simulink model "electricCar230823"  (R2020b)
settings: Solver=FixedStepAuto  StartTime=0.0  StopTime=SIMULPARAM.T_end  FixedStep=SIMULPARAM.Ts  RelTol=1e-3
undefined symbols (not defined in the file or in its folder): BAT, C, CHAp, Currentcontroller, DCM, F, Ki_Current_Con, Kp_Current_Con, Kp_Ucap, Linduc, MTp, RDp, Rinduc, Speedcontroller, T, Uco
libraries: simulink x1
settings Model: Creator=PC  LastModifiedBy=PC

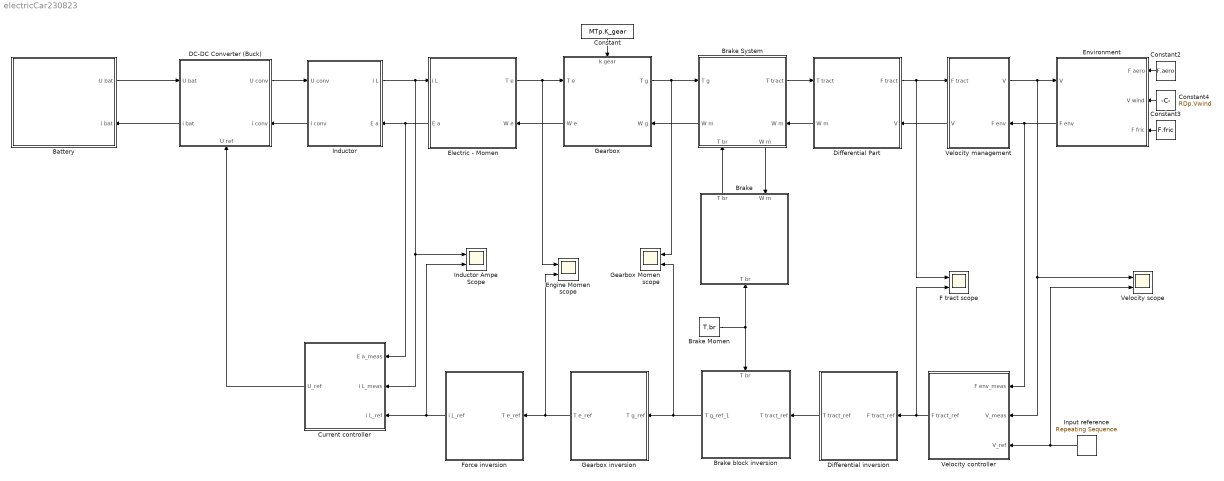
== system electricCar230823 ==
  Battery : Subsystem
      settings: PortSchema="{\"entries\":[{\"content\":{\"sides\":[{\"content\":{\"connectorIds\":[]},\"type\":\"ConnectorPlacement.EquallySpacedRectSide\",\"uuid\":\"1728278d-2efb-45d4-8f99-b2a86feaa846\"},{\"content\":{\"connectorIds\":[\"Out1\",\"In1\"],\"side\":\"RIGHT\"},\"type\":\"ConnectorPlacement.EquallySpacedRectSide\",\"uuid\":\"72e7f82c-4a4c-4bdc-a479-895fa91bb5d6\"},{\"content\":{\"connectorIds\":[],\"side\":\"TOP\"},\"type\":\"ConnectorPlacement.EquallySpacedRectSide\",\"uuid\":\"4ecd59fb-c886-47cd-9c71-6f362398ed11\"},{\"content\":{\"connectorIds\":[],\"side\":\"HIDDEN\"},\"type\":\"ConnectorPlacement.EquallySpacedRectSide\",\"uuid\":\"481497fe-ed83-4130-bda0-6381f15eb2c9\"}]},\"type\":\"ConnectorPlacement.EquallySpacedConnector\",\"uuid\":\"ea3c396a-3ef7-43d2-bef5-b2521c5226f8\"}],\"packageUris\":[\"http://schema.mathworks.com/mf0/Connector/R2020b\"],\"version\":\"1.0\"}"
      mask Display:
      | plot(0,0,100,100, 1.2*[50,57.68,60.77,63.08,64.97,66.58,68,69.26,70.4, 	71.42,72.36,78.28,80,78.28,72.36,71.42,70.4, 	69.26,68,66.58,64.97,63.08,60.77,57.68,50,42.32, 	39.23,36.92,35.03,33.42,32,30.74,29.6,28.58, 	27.64,21.72,20,21.72,27.64,28.58,29.6,30.74,32, 	33.42,35.03,36.92,39.23,42.32,50]-10, 1.2*[20,21,22,23,24,25,26,27,28,29,30,40,50,60,70,71,72, 	73,74,75,76,77,78,79,80,79,78,77,76,75,74,73,72, 	71,70,60,50,40,30,29,28,27,26,25,24,23,22,21,20]-10)
      | disp('ES')
  Brake : Subsystem
      settings: PortSchema="{\"entries\":[{\"content\":{\"sides\":[{\"content\":{\"connectorIds\":[\"In1\",\"Out1\"]},\"type\":\"ConnectorPlacement.EquallySpacedRectSide\",\"uuid\":\"1728278d-2efb-45d4-8f99-b2a86feaa846\"},{\"content\":{\"connectorIds\":[\"In2\"],\"side\":\"RIGHT\"},\"type\":\"ConnectorPlacement.EquallySpacedRectSide\",\"uuid\":\"72e7f82c-4a4c-4bdc-a479-895fa91bb5d6\"},{\"content\":{\"connectorIds\":[],\"side\":\"TOP\"},\"type\":\"ConnectorPlacement.EquallySpacedRectSide\",\"uuid\":\"4ecd59fb-c886-47cd-9c71-6f362398ed11\"},{\"content\":{\"connectorIds\":[],\"side\":\"HIDDEN\"},\"type\":\"ConnectorPlacement.EquallySpacedRectSide\",\"uuid\":\"481497fe-ed83-4130-bda0-6381f15eb2c9\"}]},\"type\":\"ConnectorPlacement.EquallySpacedConnector\",\"uuid\":\"ea3c396a-3ef7-43d2-bef5-b2521c5226f8\"}],\"packageUris\":[\"http://schema.mathworks.com/mf0/Connector/R2020b\"],\"version\":\"1.0\"}"
      mask Display:
      | plot(0,0,100,100, 1.2*[50,57.68,60.77,63.08,64.97,66.58,68,69.26,70.4, 	71.42,72.36,78.28,80,78.28,72.36,71.42,70.4, 	69.26,68,66.58,64.97,63.08,60.77,57.68,50,42.32, 	39.23,36.92,35.03,33.42,32,30.74,29.6,28.58, 	27.64,21.72,20,21.72,27.64,28.58,29.6,30.74,32, 	33.42,35.03,36.92,39.23,42.32,50]-10, 1.2*[20,21,22,23,24,25,26,27,28,29,30,40,50,60,70,71,72, 	73,74,75,76,77,78,79,80,79,78,77,76,75,74,73,72, 	71,70,60,50,40,30,29,28,27,26,25,24,23,22,21,20]-10)
      | disp('MS')
  Brake Momen : Constant  Value=T.br
  Brake System : Subsystem  mask(CM){}
      settings: PortSchema="{\"entries\":[{\"content\":{\"sides\":[{\"content\":{\"connectorIds\":[\"In1\",\"Out3\"]},\"type\":\"ConnectorPlacement.EquallySpacedRectSide\",\"uuid\":\"62bc74ff-9f0a-435b-bbdb-72403e9cc1db\"},{\"content\":{\"connectorIds\":[\"Out1\",\"In3\"],\"side\":\"RIGHT\"},\"type\":\"ConnectorPlacement.EquallySpacedRectSide\",\"uuid\":\"e16e9817-8001-4871-9942-49d69e9da80f\"},{\"content\":{\"connectorIds\":[],\"side\":\"TOP\"},\"type\":\"ConnectorPlacement.EquallySpacedRectSide\",\"uuid\":\"0e99ecee-f353-402b-98e6-e62629e3b5c0\"},{\"content\":{\"connectorIds\":[\"In2\",\"Out2\"],\"side\":\"BOTTOM\"},\"type\":\"ConnectorPlacement.EquallySpacedRectSide\",\"uuid\":\"3f9b191f-4efa-4e46-9672-1631f2ad3889\"},{\"content\":{\"connectorIds\":[],\"side\":\"HIDDEN\"},\"type\":\"ConnectorPlacement.EquallySpacedRectSide\",\"uuid\":\"eab2a9d2-f7eb-47b5-b573-a1d51d411443\"}]},\"type\":\"ConnectorPlacement.EquallySpacedConnector\",\"uuid\":\"edb337c0-73db-4b78-b52e-7735544c1492\"}],\"packageUris\":[\"http://schema.mathworks.com/mf0/Connector/R2020b\"],\"version\":\"1.0\"}"
      mask Display: plot(0,0,100,100,[35,35,95,95,35],[65,10,10,65,65], [5,5,65,65,5],[90,35,35,90,90])
  "Brake block inversion " : Subsystem
      settings: PortSchema="{\"entries\":[{\"content\":{\"sides\":[{\"content\":{\"connectorIds\":[\"In1\"]},\"type\":\"ConnectorPlacement.EquallySpacedRectSide\",\"uuid\":\"730055a7-c930-4640-a945-75cf3ba3ff6f\"},{\"content\":{\"connectorIds\":[\"Out1\"],\"side\":\"RIGHT\"},\"type\":\"ConnectorPlacement.EquallySpacedRectSide\",\"uuid\":\"ff5124cd-06d0-417f-b0e4-eab59cd93227\"},{\"content\":{\"connectorIds\":[\"In2\"],\"side\":\"TOP\"},\"type\":\"ConnectorPlacement.EquallySpacedRectSide\",\"uuid\":\"dac7e156-045e-4392-b76a-344f17dcf5dc\"},{\"content\":{\"connectorIds\":[],\"side\":\"HIDDEN\"},\"type\":\"ConnectorPlacement.EquallySpacedRectSide\",\"uuid\":\"42e29ba6-0723-44e9-ba7d-78428fe859ea\"}]},\"type\":\"ConnectorPlacement.EquallySpacedConnector\",\"uuid\":\"81c30e31-29e4-493d-8a58-533eb4e50f51\"}],\"packageUris\":[\"http://schema.mathworks.com/mf0/Connector/R2020b\"],\"version\":\"1.0\"}"
      mask Display: plot(0,0,100,100,[20,40,100,80,20],[75,20,20,75,75], [0,20,80,60,0],[85,30,30,85,85])
  Constant : Constant  Value=MTp.K_gear
  Constant2 : Constant  Value=F.aero
  Constant3 : Constant  Value=F.fric
  Constant4 : Constant  Value=RDp.Vwind
  Current controller : Subsystem
      mask Display: plot(0,0,100,100, [10,30,90,70,10,90],[90,10,10,90,90,10])
  DC-DC Converter (Buck) : Subsystem
      settings: PortSchema="{\"entries\":[{\"content\":{\"sides\":[{\"content\":{\"connectorIds\":[\"In1\",\"Out2\"]},\"type\":\"ConnectorPlacement.EquallySpacedRectSide\",\"uuid\":\"f2e25d2c-aa7f-4861-8c3a-38af6928b037\"},{\"content\":{\"connectorIds\":[\"Out1\",\"In3\"],\"side\":\"RIGHT\"},\"type\":\"ConnectorPlacement.EquallySpacedRectSide\",\"uuid\":\"82b8127f-d667-4684-9845-8beb7a647838\"},{\"content\":{\"connectorIds\":[],\"side\":\"TOP\"},\"type\":\"ConnectorPlacement.EquallySpacedRectSide\",\"uuid\":\"76c3910b-3260-4deb-ab83-4fcb3794542a\"},{\"content\":{\"connectorIds\":[\"In2\"],\"side\":\"BOTTOM\"},\"type\":\"ConnectorPlacement.EquallySpacedRectSide\",\"uuid\":\"340d5235-774f-48d9-bcc2-670650272594\"},{\"content\":{\"connectorIds\":[],\"side\":\"HIDDEN\"},\"type\":\"ConnectorPlacement.EquallySpacedRectSide\",\"uuid\":\"3b8b73f1-b23a-4cba-8ed6-bcf75c8f378e\"}]},\"type\":\"ConnectorPlacement.EquallySpacedConnector\",\"uuid\":\"8076e3c1-f844-447c-82cb-af3927bb8eb4\"}],\"packageUris\":[\"http://schema.mathworks.com/mf0/Connector/R2020b\"],\"version\":\"1.0\"}"
  Differential Part : Subsystem
      settings: PortSchema="{\"entries\":[{\"content\":{\"sides\":[{\"content\":{\"connectorIds\":[\"In1\",\"Out2\"]},\"type\":\"ConnectorPlacement.EquallySpacedRectSide\",\"uuid\":\"b394e922-8364-4918-bac2-7f5831442eb0\"},{\"content\":{\"connectorIds\":[\"Out1\",\"In2\"],\"side\":\"RIGHT\"},\"type\":\"ConnectorPlacement.EquallySpacedRectSide\",\"uuid\":\"e0445a5e-fdf7-4c21-a205-54d904cb27ed\"},{\"content\":{\"connectorIds\":[],\"side\":\"TOP\"},\"type\":\"ConnectorPlacement.EquallySpacedRectSide\",\"uuid\":\"c34109ca-a85d-4763-b4ce-c9c887f4fb15\"},{\"content\":{\"connectorIds\":[],\"side\":\"HIDDEN\"},\"type\":\"ConnectorPlacement.EquallySpacedRectSide\",\"uuid\":\"2368fea2-69ff-4966-ae44-ff953213b5b6\"}]},\"type\":\"ConnectorPlacement.EquallySpacedConnector\",\"uuid\":\"11143b87-4d9b-4f42-a2c1-62596b1f3291\"}],\"packageUris\":[\"http://schema.mathworks.com/mf0/Connector/R2020b\"],\"version\":\"1.0\"}"
      mask Display: plot(0,0,100,100, 1.4*[50,57.68,60.77,63.08,64.97,66.58,68,69.26,70.4, 	71.42,72.36,78.28,80,78.28,72.36,71.42,70.4, 	69.26,68,66.58,64.97,63.08,60.77,57.68,50,42.32, 	39.23,36.92,35.03,33.42,32,30.74,29.6,28.58, 	27.64,21.72,20,21.72,27.64,28.58,29.6,30.74,32, 	33.42,35.03,36.92,39.23,42.32,50]-20, 1.4*[20,21,22,23,24,25,26,27,28,29,30,40,50,60,70,71,72, 	73,74,75,76,77,78,79,80,79,78,77,76,75,74,73,72, 	71,70,60,50,40,30,29,28,27,26,25,24,23,22,21,20]-20)
  Differential inversion : Subsystem
      mask Display: plot(0,0,100,100,[10,30,90,70,10],[90,10,10,90,90])
  Electric - Momen : Subsystem
      settings: PortSchema="{\"entries\":[{\"content\":{\"sides\":[{\"content\":{\"connectorIds\":[\"In1\",\"Out2\"]},\"type\":\"ConnectorPlacement.EquallySpacedRectSide\",\"uuid\":\"b394e922-8364-4918-bac2-7f5831442eb0\"},{\"content\":{\"connectorIds\":[\"Out1\",\"In2\"],\"side\":\"RIGHT\"},\"type\":\"ConnectorPlacement.EquallySpacedRectSide\",\"uuid\":\"e0445a5e-fdf7-4c21-a205-54d904cb27ed\"},{\"content\":{\"connectorIds\":[],\"side\":\"TOP\"},\"type\":\"ConnectorPlacement.EquallySpacedRectSide\",\"uuid\":\"c34109ca-a85d-4763-b4ce-c9c887f4fb15\"},{\"content\":{\"connectorIds\":[],\"side\":\"HIDDEN\"},\"type\":\"ConnectorPlacement.EquallySpacedRectSide\",\"uuid\":\"2368fea2-69ff-4966-ae44-ff953213b5b6\"}]},\"type\":\"ConnectorPlacement.EquallySpacedConnector\",\"uuid\":\"11143b87-4d9b-4f42-a2c1-62596b1f3291\"}],\"packageUris\":[\"http://schema.mathworks.com/mf0/Connector/R2020b\"],\"version\":\"1.0\"}"
      mask Display: plot(0,0,100,100, 1.4*[50,57.68,60.77,63.08,64.97,66.58,68,69.26,70.4, 	71.42,72.36,78.28,80,78.28,72.36,71.42,70.4, 	69.26,68,66.58,64.97,63.08,60.77,57.68,50,42.32, 	39.23,36.92,35.03,33.42,32,30.74,29.6,28.58, 	27.64,21.72,20,21.72,27.64,28.58,29.6,30.74,32, 	33.42,35.03,36.92,39.23,42.32,50]-20, 1.4*[20,21,22,23,24,25,26,27,28,29,30,40,50,60,70,71,72, 	73,74,75,76,77,78,79,80,79,78,77,76,75,74,73,72, 	71,70,60,50,40,30,29,28,27,26,25,24,23,22,21,20]-20)
  Engine Momen scope : Scope  NumInputPorts=2
  Environment : Subsystem
      settings: PortSchema="{\"entries\":[{\"content\":{\"sides\":[{\"content\":{\"connectorIds\":[\"In1\",\"Out1\"]},\"type\":\"ConnectorPlacement.EquallySpacedRectSide\",\"uuid\":\"1728278d-2efb-45d4-8f99-b2a86feaa846\"},{\"content\":{\"connectorIds\":[\"In2\",\"In3\",\"In4\"],\"side\":\"RIGHT\"},\"type\":\"ConnectorPlacement.EquallySpacedRectSide\",\"uuid\":\"72e7f82c-4a4c-4bdc-a479-895fa91bb5d6\"},{\"content\":{\"connectorIds\":[],\"side\":\"TOP\"},\"type\":\"ConnectorPlacement.EquallySpacedRectSide\",\"uuid\":\"4ecd59fb-c886-47cd-9c71-6f362398ed11\"},{\"content\":{\"connectorIds\":[],\"side\":\"BOTTOM\"},\"type\":\"ConnectorPlacement.EquallySpacedRectSide\",\"uuid\":\"f99f3cdf-333c-494c-9d28-40c67ff9c903\"},{\"content\":{\"connectorIds\":[],\"side\":\"HIDDEN\"},\"type\":\"ConnectorPlacement.EquallySpacedRectSide\",\"uuid\":\"481497fe-ed83-4130-bda0-6381f15eb2c9\"}]},\"type\":\"ConnectorPlacement.EquallySpacedConnector\",\"uuid\":\"ea3c396a-3ef7-43d2-bef5-b2521c5226f8\"}],\"packageUris\":[\"http://schema.mathworks.com/mf0/Connector/R2020b\"],\"version\":\"1.0\"}"
      mask Display:
      | plot(0,0,100,100, 1.2*[50,57.68,60.77,63.08,64.97,66.58,68,69.26,70.4, 	71.42,72.36,78.28,80,78.28,72.36,71.42,70.4, 	69.26,68,66.58,64.97,63.08,60.77,57.68,50,42.32, 	39.23,36.92,35.03,33.42,32,30.74,29.6,28.58, 	27.64,21.72,20,21.72,27.64,28.58,29.6,30.74,32, 	33.42,35.03,36.92,39.23,42.32,50]-10, 1.2*[20,21,22,23,24,25,26,27,28,29,30,40,50,60,70,71,72, 	73,74,75,76,77,78,79,80,79,78,77,76,75,74,73,72, 	71,70,60,50,40,30,29,28,27,26,25,24,23,22,21,20]-10)
      | disp('MS')
  F tract scope : Scope  NumInputPorts=2
  Force inversion : Subsystem
      mask Display: plot(0,0,100,100,[10,30,90,70,10],[90,10,10,90,90])
  Gearbox : Subsystem  mask(Hacheur){}
      settings: PortSchema="{\"entries\":[{\"content\":{\"sides\":[{\"content\":{\"connectorIds\":[\"In1\",\"Out2\"]},\"type\":\"ConnectorPlacement.EquallySpacedRectSide\",\"uuid\":\"d88878b3-8f90-4ef1-90e8-2bd7cd7a4565\"},{\"content\":{\"connectorIds\":[\"Out1\",\"In3\"],\"side\":\"RIGHT\"},\"type\":\"ConnectorPlacement.EquallySpacedRectSide\",\"uuid\":\"d9733dfd-1e25-499b-80f7-04f083537083\"},{\"content\":{\"connectorIds\":[\"In2\"],\"side\":\"TOP\"},\"type\":\"ConnectorPlacement.EquallySpacedRectSide\",\"uuid\":\"7063ddce-722e-4bc9-ac26-cf4ab5e61559\"},{\"content\":{\"connectorIds\":[],\"side\":\"BOTTOM\"},\"type\":\"ConnectorPlacement.EquallySpacedRectSide\",\"uuid\":\"2850ab80-1d34-4652-9b8a-8e0e6fbc5749\"},{\"content\":{\"connectorIds\":[],\"side\":\"HIDDEN\"},\"type\":\"ConnectorPlacement.EquallySpacedRectSide\",\"uuid\":\"288ff06e-21e8-474f-a776-208acbd15993\"}]},\"type\":\"ConnectorPlacement.EquallySpacedConnector\",\"uuid\":\"1890fa73-b710-46d0-95bc-083b3bceb9fd\"}],\"packageUris\":[\"http://schema.mathworks.com/mf0/Connector/R2020b\"],\"version\":\"1.0\"}"
      mask Display: plot(0,0,100,100,[10,10,90,90,10],[90,10,10,90,90])
  Gearbox Momen scope : Scope  NumInputPorts=2
  Gearbox inversion : Subsystem
      mask Display: plot(0,0,100,100,[10,30,90,70,10],[90,10,10,90,90])
  Inductor : Subsystem  mask(CM){}
      settings: PortSchema="{\"entries\":[{\"content\":{\"sides\":[{\"content\":{\"connectorIds\":[\"In1\",\"Out2\"]},\"type\":\"ConnectorPlacement.EquallySpacedRectSide\",\"uuid\":\"b394e922-8364-4918-bac2-7f5831442eb0\"},{\"content\":{\"connectorIds\":[\"Out1\",\"In2\"],\"side\":\"RIGHT\"},\"type\":\"ConnectorPlacement.EquallySpacedRectSide\",\"uuid\":\"e0445a5e-fdf7-4c21-a205-54d904cb27ed\"},{\"content\":{\"connectorIds\":[],\"side\":\"TOP\"},\"type\":\"ConnectorPlacement.EquallySpacedRectSide\",\"uuid\":\"c34109ca-a85d-4763-b4ce-c9c887f4fb15\"},{\"content\":{\"connectorIds\":[],\"side\":\"HIDDEN\"},\"type\":\"ConnectorPlacement.EquallySpacedRectSide\",\"uuid\":\"2368fea2-69ff-4966-ae44-ff953213b5b6\"}]},\"type\":\"ConnectorPlacement.EquallySpacedConnector\",\"uuid\":\"11143b87-4d9b-4f42-a2c1-62596b1f3291\"}],\"packageUris\":[\"http://schema.mathworks.com/mf0/Connector/R2020b\"],\"version\":\"1.0\"}"
      mask Display: plot(0,0,100,100,[10,10,90,90,10],[90,10,10,90,90], [10,90],[10,90])
  Inductor Ampe Scope : Scope  NumInputPorts=2
  Input reference : simulink/Sources/Repeating Sequence  rep_seq_t=[0 5 10 20 50.5 66.5 107.5]  rep_seq_y=[5 0 0 30 40 40*1.5 40*1.5]
  Velocity controller : Subsystem
      mask Display: plot(0,0,100,100, [10,30,90,70,10,90],[90,10,10,90,90,10])
  Velocity management : Subsystem  mask(CM){}
      settings: PortSchema="{\"entries\":[{\"content\":{\"sides\":[{\"content\":{\"connectorIds\":[\"In1\",\"Out2\"]},\"type\":\"ConnectorPlacement.EquallySpacedRectSide\",\"uuid\":\"b394e922-8364-4918-bac2-7f5831442eb0\"},{\"content\":{\"connectorIds\":[\"Out1\",\"In2\"],\"side\":\"RIGHT\"},\"type\":\"ConnectorPlacement.EquallySpacedRectSide\",\"uuid\":\"e0445a5e-fdf7-4c21-a205-54d904cb27ed\"},{\"content\":{\"connectorIds\":[],\"side\":\"TOP\"},\"type\":\"ConnectorPlacement.EquallySpacedRectSide\",\"uuid\":\"c34109ca-a85d-4763-b4ce-c9c887f4fb15\"},{\"content\":{\"connectorIds\":[],\"side\":\"HIDDEN\"},\"type\":\"ConnectorPlacement.EquallySpacedRectSide\",\"uuid\":\"2368fea2-69ff-4966-ae44-ff953213b5b6\"}]},\"type\":\"ConnectorPlacement.EquallySpacedConnector\",\"uuid\":\"11143b87-4d9b-4f42-a2c1-62596b1f3291\"}],\"packageUris\":[\"http://schema.mathworks.com/mf0/Connector/R2020b\"],\"version\":\"1.0\"}"
      mask Display: plot(0,0,100,100,[10,10,90,90,10],[90,10,10,90,90], [10,90],[10,90])
  Velocity scope : Scope  NumInputPorts=2
  wires:
  DC-DC Converter (Buck)/1(U conv) -> Inductor/1(U conv)
  DC-DC Converter (Buck)/2(i bat) -> Battery/1(i bat)
  Constant/1 -> Gearbox/2(k gear)
  Battery/1(U bat) -> DC-DC Converter (Buck)/1(U bat)
  Electric - Momen/2(E a) -> Current controller/1(E a_meas), Inductor/2(E a)
  Inductor/1(i L) -> Inductor Ampe Scope/1, Current controller/2(i L_meas), Electric - Momen/1(i L)
  Gearbox/2(W e) -> Electric - Momen/2(W e)
  Inductor/2(i conv) -> DC-DC Converter (Buck)/3(i conv)
  Electric - Momen/1(T e) -> Engine Momen scope/1, Gearbox/1(T e)
  Brake System/2(W m) -> Brake/1(W m)
  Brake/1("T br ") -> Brake System/2(T br)
  Gearbox/1(T g) -> Brake System/1(T g), Gearbox Momen scope/1
  Brake System/3("W m  ") -> Gearbox/3(W g)
  Velocity management/2(V) -> Differential Part/2(V)
  Differential Part/1(F tract) -> F tract scope/1, Velocity management/1(F tract)
  Brake System/1(T tract) -> Differential Part/1(T tract)
  Differential Part/2(W m) -> Brake System/3("W m ")
  Environment/1(F env) -> Velocity controller/1(F env_meas), Velocity management/2(F env)
  Current controller/1(U_ref) -> DC-DC Converter (Buck)/2(U ref)
  Constant3/1 -> Environment/4(F fric)
  Constant2/1 -> Environment/2(F aero)
  Constant4/1 -> Environment/3(V wind)
  Force inversion/1(i L_ref) -> Inductor Ampe Scope/2, Current controller/3(i L_ref)
  Velocity controller/1(F tract_ref) -> F tract scope/2, Differential inversion/1(F tract_ref)
  Differential inversion/1(T tract_ref) -> "Brake block inversion "/1(T tract_ref)
  "Brake block inversion "/1(T g_ref_1) -> Gearbox Momen scope/2, Gearbox inversion/1(T g_ref)
  Gearbox inversion/1(T e_ref) -> Engine Momen scope/2, Force inversion/1(T e_ref)
  Velocity management/1("V ") -> Environment/1(V), Velocity controller/2(V_meas), Velocity scope/1
  Input reference/1 -> Velocity scope/2, Velocity controller/3(V_ref)
  Brake Momen/1 -> "Brake block inversion "/2(T br), Brake/2(T br)

== system electricCar230823/Battery ==
  i bat : Inport
  Constant : Constant  Value=BAT.U
  Terminator : Terminator
  U bat : Outport  InitialOutput=0
  wires:
  i bat/1 -> Terminator/1
  Constant/1 -> U bat/1

== system electricCar230823/Brake ==
  W m : Inport
  T br : Inport  Port=2
  Terminator : Terminator
  "T br " : Outport  InitialOutput=0
  wires:
  T br/1 -> "T br "/1
  W m/1 -> Terminator/1

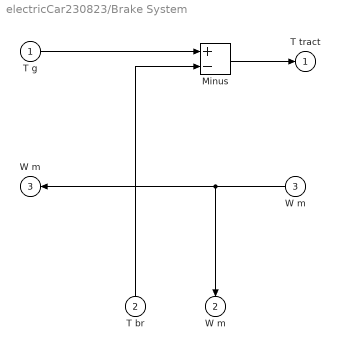
== system electricCar230823/Brake System ==
  T g : Inport
  T br : Inport  Port=2
  "W m " : Inport  Port=3
  Minus : Sum  Inputs=+-
  T tract : Outport  InitialOutput=0
  W m : Outport  Port=2  InitialOutput=0
  "W m  " : Outport  Port=3  InitialOutput=0
  wires:
  T g/1 -> Minus/1
  Minus/1 -> T tract/1
  T br/1 -> Minus/2
  "W m "/1 -> W m/1, "W m  "/1

== system electricCar230823/Brake block inversion  ==
  T tract_ref : Inport
  T br : Inport  Port=2
  Minus : Sum  Inputs=+-
  T g_ref_1 : Outport  InitialOutput=0
  wires:
  T tract_ref/1 -> Minus/1
  T br/1 -> Minus/2
  Minus/1 -> T g_ref_1/1

== system electricCar230823/Current controller ==
  E a_meas : Inport
  i L_meas : Inport  Port=2
  i L_ref : Inport  Port=3
  IP Controller : Subsystem
  PI Controller : Subsystem
  U_ref : Outport  InitialOutput=0
  wires:
  PI Controller/1(U_ref) -> U_ref/1
  i L_meas/1 -> PI Controller/2(i L_meas)
  E a_meas/1 -> PI Controller/1(E a_meas)
  i L_ref/1 -> PI Controller/3(i L_ref)

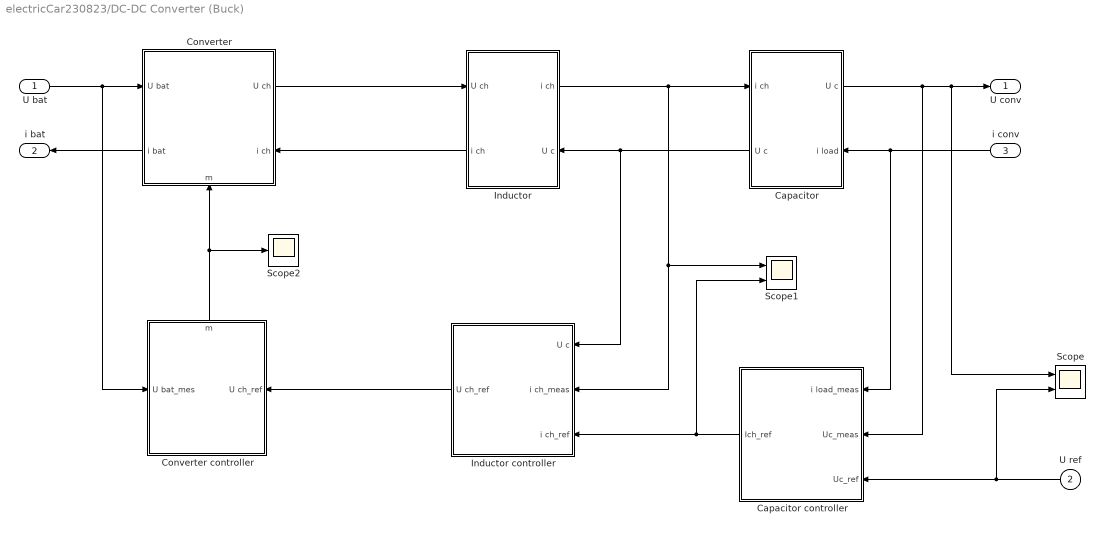
== system electricCar230823/DC-DC Converter (Buck) ==
  U bat : Inport
  U ref : Inport  Port=2
  i conv : Inport  Port=3
  Capacitor : Subsystem  mask(CM){}
      settings: PortSchema="{\"entries\":[{\"content\":{\"sides\":[{\"content\":{\"connectorIds\":[\"In1\",\"Out2\"]},\"type\":\"ConnectorPlacement.EquallySpacedRectSide\",\"uuid\":\"8b9f6a53-b0ce-4fb6-ba22-844cc3c0ad7c\"},{\"content\":{\"connectorIds\":[\"Out1\",\"In2\"],\"side\":\"RIGHT\"},\"type\":\"ConnectorPlacement.EquallySpacedRectSide\",\"uuid\":\"cf1dddcb-91a5-42be-b809-81485d04749f\"},{\"content\":{\"connectorIds\":[],\"side\":\"TOP\"},\"type\":\"ConnectorPlacement.EquallySpacedRectSide\",\"uuid\":\"6b0fe42a-e78b-443e-b09d-31143c938294\"},{\"content\":{\"connectorIds\":[],\"side\":\"HIDDEN\"},\"type\":\"ConnectorPlacement.EquallySpacedRectSide\",\"uuid\":\"92c1545a-c508-44c0-b705-53a96b01068d\"}]},\"type\":\"ConnectorPlacement.EquallySpacedConnector\",\"uuid\":\"979f83f8-9940-4886-be45-d6e0e0e53bbd\"}],\"packageUris\":[\"http://schema.mathworks.com/mf0/Connector/R2020b\"],\"version\":\"1.0\"}"
      mask Display: plot(0,0,100,100,[10,10,90,90,10],[90,10,10,90,90], [10,90],[10,90])
  Capacitor controller : Subsystem
      mask Display: plot(0,0,100,100, [10,30,90,70,10,90],[90,10,10,90,90,10])
  Converter : Subsystem  mask(Hacheur){}
      settings: PortSchema="{\"entries\":[{\"content\":{\"sides\":[{\"content\":{\"connectorIds\":[\"In1\",\"Out2\"]},\"type\":\"ConnectorPlacement.EquallySpacedRectSide\",\"uuid\":\"c60d43d5-6da5-438e-89cb-fd4b71327869\"},{\"content\":{\"connectorIds\":[\"Out1\",\"In3\"],\"side\":\"RIGHT\"},\"type\":\"ConnectorPlacement.EquallySpacedRectSide\",\"uuid\":\"3d284952-b10a-4f69-b6ba-c89d88fd27ff\"},{\"content\":{\"connectorIds\":[],\"side\":\"TOP\"},\"type\":\"ConnectorPlacement.EquallySpacedRectSide\",\"uuid\":\"b76f213b-a89b-4ddb-95af-c15166783b82\"},{\"content\":{\"connectorIds\":[\"In2\"],\"side\":\"BOTTOM\"},\"type\":\"ConnectorPlacement.EquallySpacedRectSide\",\"uuid\":\"5563bba7-a4d6-45e0-a571-46d0680df108\"},{\"content\":{\"connectorIds\":[],\"side\":\"HIDDEN\"},\"type\":\"ConnectorPlacement.EquallySpacedRectSide\",\"uuid\":\"086c2170-6f4c-4142-a25f-314308635861\"}]},\"type\":\"ConnectorPlacement.EquallySpacedConnector\",\"uuid\":\"18a4dcbf-0877-4e56-9ceb-c80d259dd4b7\"}],\"packageUris\":[\"http://schema.mathworks.com/mf0/Connector/R2020b\"],\"version\":\"1.0\"}"
      mask Display: plot(0,0,100,100,[10,10,90,90,10],[90,10,10,90,90])
  Converter controller : Subsystem
      settings: PortSchema="{\"entries\":[{\"content\":{\"sides\":[{\"content\":{\"connectorIds\":[\"In1\"]},\"type\":\"ConnectorPlacement.EquallySpacedRectSide\",\"uuid\":\"badc3caa-6192-4446-bf39-33dbdad74a9c\"},{\"content\":{\"connectorIds\":[\"In2\"],\"side\":\"RIGHT\"},\"type\":\"ConnectorPlacement.EquallySpacedRectSide\",\"uuid\":\"1170bffd-3f0f-42f5-893b-0e18c3005bf1\"},{\"content\":{\"connectorIds\":[\"Out1\"],\"side\":\"TOP\"},\"type\":\"ConnectorPlacement.EquallySpacedRectSide\",\"uuid\":\"7a85b726-b466-447a-a747-1454cd7b1f05\"},{\"content\":{\"connectorIds\":[],\"side\":\"HIDDEN\"},\"type\":\"ConnectorPlacement.EquallySpacedRectSide\",\"uuid\":\"d7fbd796-8c34-4fc1-83a8-47ced3c788b9\"}]},\"type\":\"ConnectorPlacement.EquallySpacedConnector\",\"uuid\":\"74fa73a9-ee93-4918-a076-3243bad27dc9\"}],\"packageUris\":[\"http://schema.mathworks.com/mf0/Connector/R2020b\"],\"version\":\"1.0\"}"
      mask Display: plot(0,0,100,100,[10,30,90,70,10],[90,10,10,90,90])
  Inductor : Subsystem  mask(CM){}
      settings: PortSchema="{\"entries\":[{\"content\":{\"sides\":[{\"content\":{\"connectorIds\":[\"In1\",\"Out2\"]},\"type\":\"ConnectorPlacement.EquallySpacedRectSide\",\"uuid\":\"8b9f6a53-b0ce-4fb6-ba22-844cc3c0ad7c\"},{\"content\":{\"connectorIds\":[\"Out1\",\"In2\"],\"side\":\"RIGHT\"},\"type\":\"ConnectorPlacement.EquallySpacedRectSide\",\"uuid\":\"cf1dddcb-91a5-42be-b809-81485d04749f\"},{\"content\":{\"connectorIds\":[],\"side\":\"TOP\"},\"type\":\"ConnectorPlacement.EquallySpacedRectSide\",\"uuid\":\"6b0fe42a-e78b-443e-b09d-31143c938294\"},{\"content\":{\"connectorIds\":[],\"side\":\"HIDDEN\"},\"type\":\"ConnectorPlacement.EquallySpacedRectSide\",\"uuid\":\"92c1545a-c508-44c0-b705-53a96b01068d\"}]},\"type\":\"ConnectorPlacement.EquallySpacedConnector\",\"uuid\":\"979f83f8-9940-4886-be45-d6e0e0e53bbd\"}],\"packageUris\":[\"http://schema.mathworks.com/mf0/Connector/R2020b\"],\"version\":\"1.0\"}"
      mask Display: plot(0,0,100,100,[10,10,90,90,10],[90,10,10,90,90], [10,90],[10,90])
  Inductor controller : Subsystem
      mask Display: plot(0,0,100,100, [10,30,90,70,10,90],[90,10,10,90,90,10])
  Scope : Scope  NumInputPorts=2
  Scope1 : Scope  NumInputPorts=2
  Scope2 : Scope
  U conv : Outport
  i bat : Outport  Port=2
  wires:
  Capacitor controller/1(Ich_ref) -> Scope1/2, Inductor controller/3(i ch_ref)
  U bat/1 -> Converter controller/2(U bat_mes), Converter/1(U bat)
  Converter controller/1(m) -> Scope2/1, Converter/2(m)
  i conv/1 -> Capacitor controller/1(i load_meas), Capacitor/2(i load)
  U ref/1 -> Scope/2, Capacitor controller/3(Uc_ref)
  Inductor controller/1(U ch_ref) -> Converter controller/1(U ch_ref)
  Converter/1(U ch) -> Inductor/1(U ch)
  Capacitor/1("U c ") -> Capacitor controller/2(Uc_meas), U conv/1, Scope/1
  Converter/2(i bat) -> i bat/1
  Capacitor/2(U c) -> Inductor controller/1(U c), Inductor/2(U c)
  Inductor/2("i ch ") -> Converter/3(i ch)
  Inductor/1(i ch) -> Inductor controller/2(i ch_meas), Scope1/1, Capacitor/1(i ch)

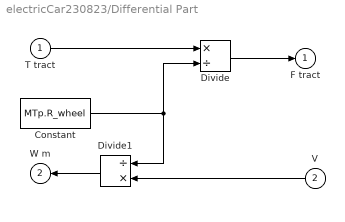
== system electricCar230823/Differential Part ==
  T tract : Inport
  V : Inport  Port=2
  Constant : Constant  Value=MTp.R_wheel
  Divide : Product  Inputs=*/
  Divide1 : Product  Inputs=/*
  F tract : Outport  InitialOutput=0
  W m : Outport  Port=2  InitialOutput=0
  wires:
  T tract/1 -> Divide/1
  Divide/1 -> F tract/1
  Divide1/1 -> W m/1
  Constant/1 -> Divide1/1, Divide/2
  V/1 -> Divide1/2

== system electricCar230823/Differential inversion ==
  F tract_ref : Inport
  Constant : Constant  Value=MTp.R_wheel
  Product : Product
  T tract_ref : Outport  InitialOutput=0
  wires:
  Product/1 -> T tract_ref/1
  F tract_ref/1 -> Product/2
  Constant/1 -> Product/1

== system electricCar230823/Electric - Momen ==
  i L : Inport
  W e : Inport  Port=2
  Gain : Gain  Gain=DCM.Kphi
  Gain1 : Gain  Gain=DCM.Kphi
  T e : Outport  InitialOutput=0
  E a : Outport  Port=2  InitialOutput=0
  wires:
  i L/1 -> Gain/1
  Gain/1 -> T e/1
  W e/1 -> Gain1/1
  Gain1/1 -> E a/1

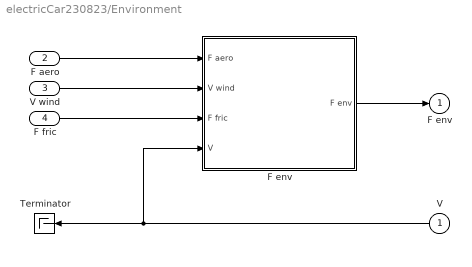
== system electricCar230823/Environment ==
  V : Inport
  F aero : Inport  Port=2
  V wind : Inport  Port=3
  F fric : Inport  Port=4
  "F env " : Subsystem
  Terminator : Terminator
  F env : Outport  InitialOutput=0
  wires:
  V/1 -> "F env "/4(V), Terminator/1
  "F env "/1(F env) -> F env/1
  F fric/1 -> "F env "/3(F fric)
  V wind/1 -> "F env "/2(V wind)
  F aero/1 -> "F env "/1(F aero)

== system electricCar230823/Force inversion ==
  T e_ref : Inport
  Constant : Constant  Value=DCM.Kphi
  Divide : Product  Inputs=*/
  i L_ref : Outport  InitialOutput=0
  wires:
  Divide/1 -> i L_ref/1
  T e_ref/1 -> Divide/1
  Constant/1 -> Divide/2

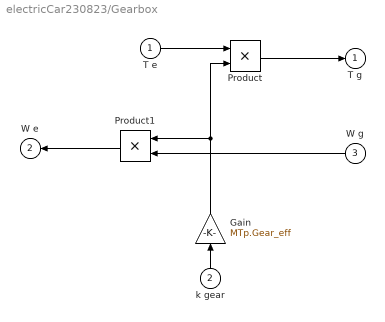
== system electricCar230823/Gearbox ==
  T e : Inport
  k gear : Inport  Port=2
  W g : Inport  Port=3
  Gain : Gain  Gain=MTp.Gear_eff
  Product : Product
  Product1 : Product
  T g : Outport  InitialOutput=0
  W e : Outport  Port=2  InitialOutput=0
  wires:
  k gear/1 -> Gain/1
  T e/1 -> Product/1
  Product/1 -> T g/1
  Gain/1 -> Product/2, Product1/1
  Product1/1 -> W e/1
  W g/1 -> Product1/2

== system electricCar230823/Gearbox inversion ==
  T g_ref : Inport
  Constant : Constant  Value=MTp.Gear_eff
  Constant1 : Constant  Value=MTp.K_gear
  Divide : Product  Inputs=*/
  Product1 : Product
  T e_ref : Outport  InitialOutput=0
  wires:
  Divide/1 -> T e_ref/1
  Constant1/1 -> Product1/2
  Constant/1 -> Product1/1
  Product1/1 -> Divide/2
  T g_ref/1 -> Divide/1

== system electricCar230823/Inductor ==
  U conv : Inport
  E a : Inport  Port=2
  Minus : Sum  Inputs=+-
  Transfer Fcn : TransferFcn  Denominator=[DCM.L DCM.R]
  i L : Outport  InitialOutput=0
  i conv : Outport  Port=2  InitialOutput=0
  wires:
  U conv/1 -> Minus/1
  E a/1 -> Minus/2
  Minus/1 -> Transfer Fcn/1
  Transfer Fcn/1 -> i conv/1, i L/1

== system electricCar230823/Velocity controller ==
  F env_meas : Inport
  V_meas : Inport  Port=2
  V_ref : Inport  Port=3
  IP Controller : Subsystem
  PI Controller : Subsystem
  F tract_ref : Outport  InitialOutput=0
  wires:
  IP Controller/1(F tract_ref) -> F tract_ref/1
  V_meas/1 -> IP Controller/2(V_meas)
  F env_meas/1 -> IP Controller/1(F env_meas)
  V_ref/1 -> IP Controller/3(V_ref)

== system electricCar230823/Velocity management ==
  F tract : Inport
  F env : Inport  Port=2
  Gain : Gain  Gain=1/CHAp.M_eq
  Integrator : Integrator
  Minus : Sum  Inputs=+-
  "V " : Outport  InitialOutput=0
  V : Outport  Port=2  InitialOutput=0
  wires:
  F tract/1 -> Minus/1
  F env/1 -> Minus/2
  Minus/1 -> Integrator/1
  Integrator/1 -> Gain/1
  Gain/1 -> V/1, "V "/1

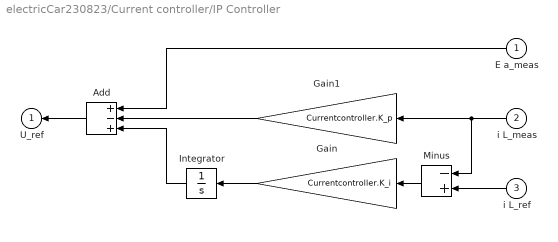
== system electricCar230823/Current controller/IP Controller ==
  E a_meas : Inport
  i L_meas : Inport  Port=2
  i L_ref : Inport  Port=3
  Add : Sum  Inputs=+-+
  Gain : Gain  Gain=Currentcontroller.K_i
  Gain1 : Gain  Gain=Currentcontroller.K_p
  Integrator : Integrator
  Minus : Sum  Inputs=-+
  U_ref : Outport  InitialOutput=0
  wires:
  Integrator/1 -> Add/3
  Gain1/1 -> Add/2
  Gain/1 -> Integrator/1
  i L_meas/1 -> Gain1/1, Minus/1
  E a_meas/1 -> Add/1
  i L_ref/1 -> Minus/2
  Add/1 -> U_ref/1
  Minus/1 -> Gain/1

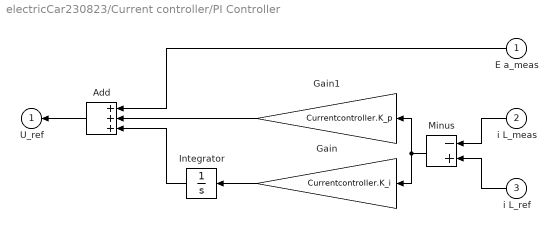
== system electricCar230823/Current controller/PI Controller ==
  E a_meas : Inport
  i L_meas : Inport  Port=2
  i L_ref : Inport  Port=3
  Add : Sum  Inputs=+++
  Gain : Gain  Gain=Currentcontroller.K_i
  Gain1 : Gain  Gain=Currentcontroller.K_p
  Integrator : Integrator
  Minus : Sum  Inputs=-+
  U_ref : Outport  InitialOutput=0
  wires:
  Integrator/1 -> Add/3
  Gain1/1 -> Add/2
  Gain/1 -> Integrator/1
  i L_meas/1 -> Minus/1
  E a_meas/1 -> Add/1
  i L_ref/1 -> Minus/2
  Add/1 -> U_ref/1
  Minus/1 -> Gain/1, Gain1/1

== system electricCar230823/DC-DC Converter (Buck)/Capacitor ==
  i ch : Inport
  i load : Inport  Port=2
  Gain : Gain  Gain=1/C
  Integrator : Integrator  InitialCondition=Uco
  Minus : Sum  Inputs=+-
  "U c " : Outport  InitialOutput=0
  U c : Outport  Port=2  InitialOutput=0
  wires:
  i ch/1 -> Minus/1
  i load/1 -> Minus/2
  Minus/1 -> Gain/1
  Gain/1 -> Integrator/1
  Integrator/1 -> "U c "/1, U c/1

== system electricCar230823/DC-DC Converter (Buck)/Capacitor controller ==
  i load_meas : Inport
  Uc_meas : Inport  Port=2
  Uc_ref : Inport  Port=3
  Gain : Gain  Gain=Kp_Ucap
  Minus : Sum  Inputs=-+
  Minus1 : Sum
  Ich_ref : Outport  InitialOutput=0
  wires:
  Uc_meas/1 -> Minus/1
  Uc_ref/1 -> Minus/2
  Minus/1 -> Gain/1
  i load_meas/1 -> Minus1/1
  Gain/1 -> Minus1/2
  Minus1/1 -> Ich_ref/1

== system electricCar230823/DC-DC Converter (Buck)/Converter ==
  U bat : Inport
  m : Inport  Port=2
  i ch : Inport  Port=3
  Product : Product
  Product1 : Product
  U ch : Outport  InitialOutput=0
  i bat : Outport  Port=2  InitialOutput=0
  wires:
  m/1 -> Product/2, Product1/2
  U bat/1 -> Product/1
  Product/1 -> U ch/1
  i ch/1 -> Product1/1
  Product1/1 -> i bat/1

== system electricCar230823/DC-DC Converter (Buck)/Converter controller ==
  U ch_ref : Inport
  U bat_mes : Inport  Port=2
  Divide : Product  Inputs=/*
  m : Outport  InitialOutput=0
  wires:
  U ch_ref/1 -> Divide/2
  U bat_mes/1 -> Divide/1
  Divide/1 -> m/1

== system electricCar230823/DC-DC Converter (Buck)/Inductor ==
  U ch : Inport
  U c : Inport  Port=2
  Minus : Sum  Inputs=+-
  Transfer Fcn : TransferFcn  Denominator=[Linduc Rinduc]
  i ch : Outport  InitialOutput=0
  "i ch " : Outport  Port=2  InitialOutput=0
  wires:
  U ch/1 -> Minus/1
  U c/1 -> Minus/2
  Minus/1 -> Transfer Fcn/1
  Transfer Fcn/1 -> i ch/1, "i ch "/1

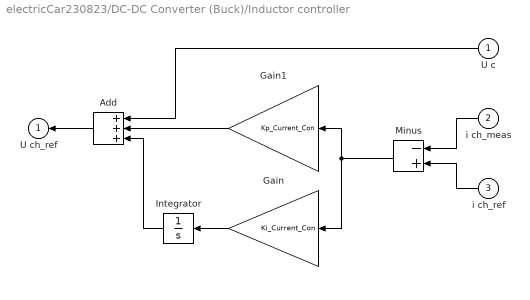
== system electricCar230823/DC-DC Converter (Buck)/Inductor controller ==
  U c : Inport
  i ch_meas : Inport  Port=2
  i ch_ref : Inport  Port=3
  Add : Sum  Inputs=+++
  Gain : Gain  Gain=Ki_Current_Con
  Gain1 : Gain  Gain=Kp_Current_Con
  Integrator : Integrator
  Minus : Sum  Inputs=-+
  U ch_ref : Outport  InitialOutput=0
  wires:
  i ch_ref/1 -> Minus/2
  i ch_meas/1 -> Minus/1
  Minus/1 -> Gain/1, Gain1/1
  Gain/1 -> Integrator/1
  Integrator/1 -> Add/3
  Gain1/1 -> Add/2
  U c/1 -> Add/1
  Add/1 -> U ch_ref/1

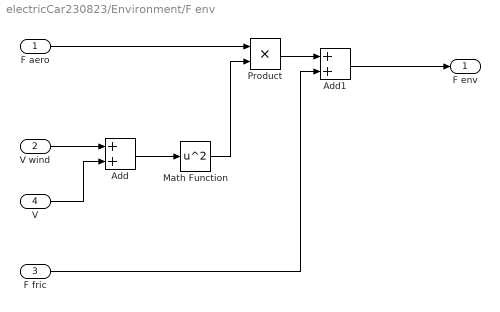
== system electricCar230823/Environment/F env  ==
  F aero : Inport
  V wind : Inport  Port=2
  F fric : Inport  Port=3
  V : Inport  Port=4
  Add : Sum
  Add1 : Sum
  Math Function : Math  Operator=square  SaturateOnIntegerOverflow=on
  Product : Product
  F env : Outport
  wires:
  V wind/1 -> Add/1
  V/1 -> Add/2
  Add/1 -> Math Function/1
  F aero/1 -> Product/1
  Math Function/1 -> Product/2
  Product/1 -> Add1/1
  F fric/1 -> Add1/2
  Add1/1 -> F env/1

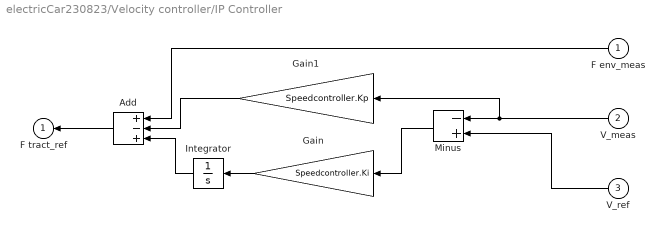
== system electricCar230823/Velocity controller/IP Controller ==
  F env_meas : Inport
  V_meas : Inport  Port=2
  V_ref : Inport  Port=3
  Add : Sum  Inputs=+-+
  Gain : Gain  Gain=Speedcontroller.Ki
  Gain1 : Gain  Gain=Speedcontroller.Kp
  Integrator : Integrator
  Minus : Sum  Inputs=-+
  F tract_ref : Outport  InitialOutput=0
  wires:
  Gain/1 -> Integrator/1
  Add/1 -> F tract_ref/1
  Gain1/1 -> Add/2
  V_ref/1 -> Minus/2
  Minus/1 -> Gain/1
  Integrator/1 -> Add/3
  F env_meas/1 -> Add/1
  V_meas/1 -> Gain1/1, Minus/1

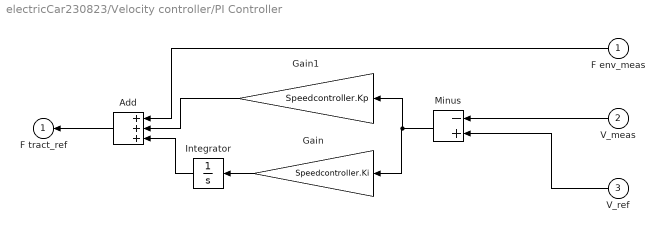
== system electricCar230823/Velocity controller/PI Controller ==
  F env_meas : Inport
  V_meas : Inport  Port=2
  V_ref : Inport  Port=3
  Add : Sum  Inputs=+++
  Gain : Gain  Gain=Speedcontroller.Ki
  Gain1 : Gain  Gain=Speedcontroller.Kp
  Integrator : Integrator
  Minus : Sum  Inputs=-+
  F tract_ref : Outport  InitialOutput=0
  wires:
  Gain/1 -> Integrator/1
  Add/1 -> F tract_ref/1
  Gain1/1 -> Add/2
  V_ref/1 -> Minus/2
  Minus/1 -> Gain1/1, Gain/1
  Integrator/1 -> Add/3
  F env_meas/1 -> Add/1
  V_meas/1 -> Minus/1
